simulink model "BLDCmotorControl_FOC_R2017b"  (R2017b)
settings: Solver=FixedStepDiscrete  StartTime=0  StopTime=1  FixedStep=Ts  MaxStep=1e-6  RelTol=1e-6  AbsTol=1e-6  EnableMultiTasking=on
PreLoadFcn:
  | addpath(genpath('01_Libraries'));
  | addpath(genpath('02_Figures'));
InitFcn:
  | init_model;
values from neighbouring files (symbols this model uses):
  a_elecAngle = 60    [init_model_Ffwd.m]
  a_elecPeriod = 360    [init_model_Ffwd.m]
  b_DCLinkCurrAvail = 0    [init_model_Ffwd.m]
  b_selPhaABCurrMeas = 1    [init_model_Ffwd.m]
  cf_speedCoef = round(f_ctrl * a_mechAngle * (pi/180) * (30/pi))    [init_model_Ffwd.m]
  i_thresOutlier = 200    [init_model_Ffwd.m]
  n_commAcvLo = 15    [init_model_Ffwd.m]
  n_commDeacvHi = 30    [init_model_Ffwd.m]
  r_sin_M1 = sin((a_elecAngle_XA + 30)*(pi/180))    [init_model_Ffwd.m]
  r_whl = 6.5 * 2.54 * 1e-2 / 2    (= 0.08255)    [init_model_Ffwd.m]
  res_elecAngle = 2    [init_model_Ffwd.m]
  Ts = 5e-6    (= 5e-06)    [init_model_Ffwd.m]    (also in pe_electric_engine_dyno_data.m = 1e-05)
  Ts_ctrl = 6e-5    (= 6e-05)    [init_model_Ffwd.m]
  vec_hallToPos = [0 2 0 1 4 3 5 0]    [init_model_Ffwd.m]
  z_commutMap_M1 = [-1 -1  0  1  1  0 ... (first row only)    [init_model_Ffwd.m]
  z_ctrlTypSel = 1    [init_model_Ffwd.m]
  z_maxCntRst = 2000    [init_model_Ffwd.m]
undefined symbols (not defined in the file or in its folder): a_phaAdv_M1, b_phaAdvEna, CTRL_COMM, DiscIntNeverNeededParam, Down, dz_counterHi, dz_counterLo, Kb_Id, Kb_Iq, Kb_n, Ki_Id, Ki_Iq, Ki_n, Kp_Id, Kp_Iq, Kp_n, n_motPhaAdvEna, r_commDCDeacv, sigbuilder_block, Up, V_circleLim_M1, V_max, V_min
libraries: pePwmGenerator x7, BLDC_controller_Lib x6, powerlib x6, simulink x5
(part 2 of 3)

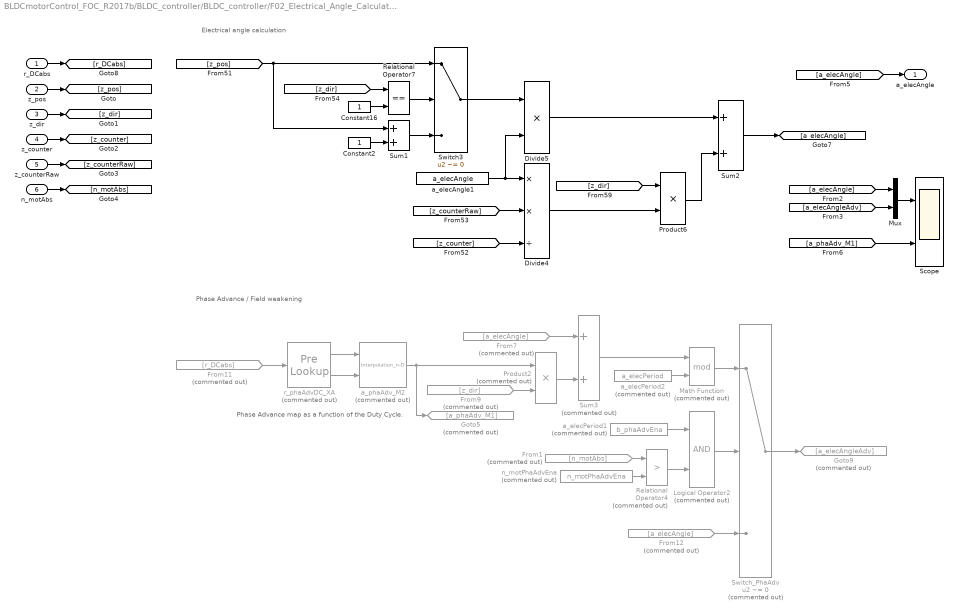
== system BLDCmotorControl_FOC_R2017b/BLDC_controller/BLDC_controller/F02_Electrical_Angle_Calculation ==
  note: Electrical angle calculation
  note: Phase Advance / Field weakening
  note: Phase Advance map as a function of the Duty Cycle.
  r_DCabs : Inport
  z_pos : Inport  Port=2
  z_dir : Inport  Port=3
  z_counter : Inport  Port=4
  z_counterRaw : Inport  Port=5
  n_motAbs : Inport  Port=6
  Constant16 : Constant  OutDataTypeStr=Inherit: Inherit via back propagation
  Constant2 : Constant  OutDataTypeStr=Inherit: Inherit via back propagation
  Divide4 : Product  Inputs=**/  OutDataTypeStr=int32  RndMeth=Simplest
  Divide5 : Product  Inputs=**  OutDataTypeStr=int32  RndMeth=Simplest
  From1 : From  Commented=on  GotoTag=n_motAbs
  From11 : From  Commented=on  GotoTag=r_DCabs
  From12 : From  Commented=on  GotoTag=a_elecAngle
  From7 : From  Commented=on  GotoTag=a_elecAngle
  From9 : From  Commented=on  GotoTag=z_dir
  Goto5 : Goto  Commented=on  GotoTag=a_phaAdv_M1
  Goto9 : Goto  Commented=on  GotoTag=a_elecAngleAdv
  Logical Operator2 : Logic  Commented=on  AllPortsSameDT=off  OutDataTypeStr=boolean
  Math Function : Math  Commented=on  Operator=mod  SaturateOnIntegerOverflow=on
  Mux : Mux  Inputs=2
  Product2 : Product  Commented=on  RndMeth=Simplest  OutDataTypeStr=Inherit: Same as first input
  Product6 : Product  OutDataTypeStr=Inherit: Inherit via back propagation  RndMeth=Simplest
  Relational Operator4 : RelationalOperator  Commented=on  Operator=>  OutDataTypeStr=boolean  RndMeth=Simplest
  Relational Operator7 : RelationalOperator  Operator===  OutDataTypeStr=boolean  RndMeth=Simplest
  Scope : Scope  NumInputPorts=2
  Sum1 : Sum  RndMeth=Simplest  OutDataTypeStr=Inherit: Same as first input
  Sum2 : Sum  RndMeth=Simplest  OutDataTypeStr=Inherit: Same as first input
  Sum3 : Sum  Commented=on  RndMeth=Simplest  OutDataTypeStr=Inherit: Same as first input
  Switch3 : Switch  Criteria=u2 ~= 0  OutDataTypeStr=Inherit: Inherit via back propagation  RndMeth=Zero
  Switch_PhaAdv : Switch  Commented=on  Criteria=u2 ~= 0  OutDataTypeStr=Inherit: Inherit via back propagation  RndMeth=Zero
  a_elecAngle1 : Constant  Value=a_elecAngle  OutDataTypeStr=int32
  a_elecPeriod1 : Constant  Commented=on  Value=b_phaAdvEna  OutDataTypeStr=boolean
  a_elecPeriod2 : Constant  Commented=on  Value=a_elecPeriod  OutDataTypeStr=Inherit: Inherit via back propagation
  a_phaAdv_M2 : Interpolation_n-D  Commented=on  NumberOfTableDimensions=1  Table=a_phaAdv_M1  ExtrapMethod=Clip  OutDataTypeStr=int16  InternalRulePriority=Speed  RndMeth=Simplest
      settings: InputPortMap=u0,u1
  n_motPhaAdvEna : Constant  Commented=on  Value=n_motPhaAdvEna  OutDataTypeStr=Inherit: Inherit via back propagation
  r_phaAdvDC_XA : PreLookup  Commented=on  BreakpointsData=r_phaAdvDC_XA  IndexSearchMethod=Evenly spaced points  BeginIndexSearchUsingPreviousIndexResult=on  IndexDataTypeStr=uint8  RndMeth=Simplest
  a_elecAngle : Outport  OutputWhenDisabled=reset  InitialOutput=0
  wires:
  a_phaAdv_M2/1 -> Goto5/1, Product2/1
  From9/1 -> Product2/2
  z_pos/1 -> [z_pos]
  z_dir/1 -> [z_dir]
  Mux/1 -> Scope/1
  [a_elecAngle] -> Mux/1
  [a_elecAngleAdv] -> Mux/2
  [a_elecAngle] -> a_elecAngle/1
  [a_phaAdv_M1] -> Scope/2
  r_phaAdvDC_XA/2 -> a_phaAdv_M2/2
  r_phaAdvDC_XA/1 -> a_phaAdv_M2/1
  From12/1 -> Switch_PhaAdv/3
  r_DCabs/1 -> [r_DCabs]
  Switch_PhaAdv/1 -> Goto9/1
  Product2/1 -> Sum3/2
  From7/1 -> Sum3/1
  From11/1 -> r_phaAdvDC_XA/1
  a_elecPeriod2/1 -> Math Function/2
  Math Function/1 -> Switch_PhaAdv/1
  Sum3/1 -> Math Function/1
  z_counterRaw/1 -> [z_counterRaw]
  z_counter/1 -> [z_counter]
  [z_counterRaw] -> Divide4/2
  Switch3/1 -> Divide5/1
  [z_dir] -> Product6/1
  Sum2/1 -> [a_elecAngle]
  [z_pos] -> Switch3/1, Sum1/1
  Constant2/1 -> Sum1/2
  [z_counter] -> Divide4/3
  Product6/1 -> Sum2/2
  Relational Operator7/1 -> Switch3/2
  Constant16/1 -> Relational Operator7/2
  a_elecAngle1/1 -> Divide5/2, Divide4/1
  [z_dir] -> Relational Operator7/1
  Sum1/1 -> Switch3/3
  Divide4/1 -> Product6/2
  Divide5/1 -> Sum2/1
  a_elecPeriod1/1 -> Logical Operator2/1
  n_motPhaAdvEna/1 -> Relational Operator4/2
  From1/1 -> Relational Operator4/1
  Relational Operator4/1 -> Logical Operator2/2
  Logical Operator2/1 -> Switch_PhaAdv/2
  n_motAbs/1 -> [n_motAbs]

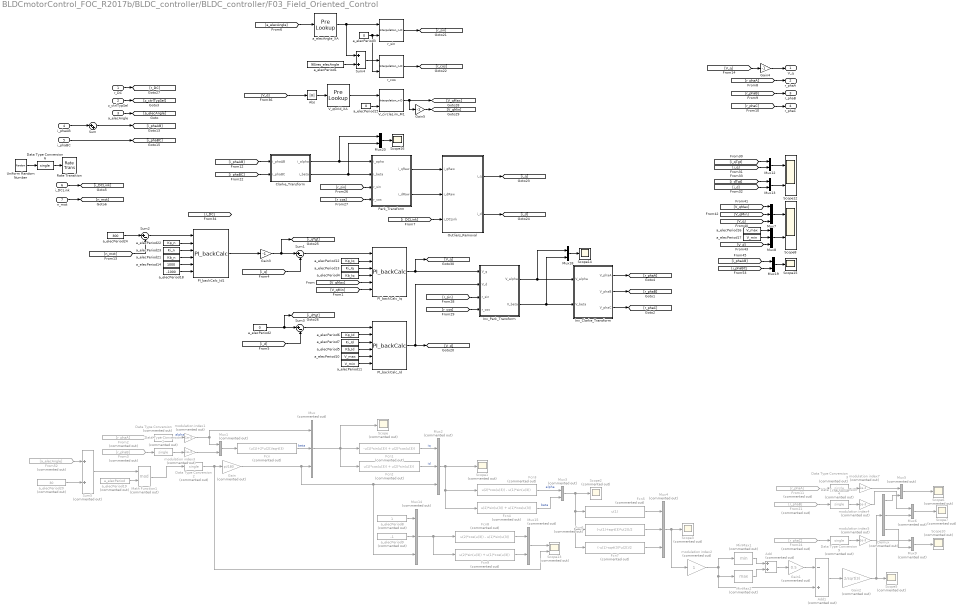
== system BLDCmotorControl_FOC_R2017b/BLDC_controller/BLDC_controller/F03_Field_Oriented_Control ==
  r_DC : Inport
  z_ctrlTypSel : Inport  Port=2
  a_elecAngle : Inport  Port=3
  i_phaAB : Inport  Port=4
  i_phaBC : Inport  Port=5
  i_DCLink : Inport  Port=6
  n_mot : Inport  Port=7
  Abs : Abs
  Add : Sum  Commented=on
  Add1 : Sum  Commented=on  Inputs=-+
  Clarke_Transform : Subsystem
  Data Type Conversion{,1..4,9} (6 alike) : DataTypeConversion  Commented=on  OutDataTypeStr=single
  Data Type Conversion6 : DataTypeConversion  OutDataTypeStr=single
  Demux : Demux  Commented=on  Outputs=3
  Fcn : Fcn  Commented=on  Expr=(u(1)+2*u(2))/sqrt(3)
  Fcn1 : Fcn  Commented=on  Expr=-u(1)*sin(u(3)) + u(2)*cos(u(3))
  Fcn2 : Fcn  Commented=on  Expr=u(1)*cos(u(3)) + u(2)*sin(u(3))
  Fcn3 : Fcn  Commented=on  Expr=u(2)*cos(u(3)) - u(1)*sin(u(3))
  Fcn4 : Fcn  Commented=on  Expr=u(2)*sin(u(3)) + u(1)*cos(u(3))
  Fcn5 : Fcn  Commented=on  Expr=u(1)
  Fcn6 : Fcn  Commented=on  Expr=(-u(1)+sqrt(3)*u(2))/2
  Fcn7 : Fcn  Commented=on  Expr=(-u(1)-sqrt(3)*u(2))/2
  Fcn8 : Fcn  Commented=on  Expr=u(2)*cos(u(3)) - u(1)*sin(u(3))
  Fcn9 : Fcn  Commented=on  Expr=u(2)*sin(u(3)) + u(1)*cos(u(3))
  From11 : From  Commented=on  GotoTag=r_phaA
  From2 : From  Commented=on  GotoTag=r_phaA
  From21 : From  Commented=on  GotoTag=r_phaB
  From24 : From  Commented=on  GotoTag=r_phaC
  From3 : From  Commented=on  GotoTag=r_phaB
  From52 : From  Commented=on  GotoTag=a_elecAngle
  Gain : Gain  Tag=struct('comment',struct('text','','placement',1),'logdata',struct('maxnumvals',inf,'plotchannels',[],'loggingmode',3,'channels',1),'output',struct('variable','','description','','name','$S_$B','width',1,'address','','max',NaN,'min',NaN,'class','default','type','CONTINUOUS','scaling','','lsb',1,'offset',0,'arb',0,'freeze',1,'unit','','autoscalingmode',1,'lowerheadroom',1,'upperheadroom',1,'headroomunit','bit','keepdatatype',1,'checkmin',0,'checkmax',0,'castoutput',0,'show',0),'gain',struct('variable','','description','','name','$S_$B_gain','width',1,'address','','max',NaN,'min',NaN,'class','default','type','CONTINUOUS','scaling','','lsb',1,'offset',0,'arb',0,'freeze',1,'unit','','keepdatatype',1,'value','1','scalar',0,'tolerance',1),'scalingvalid',0,'date',730486)  Commented=on  Gain=pi/180  RndMeth=Zero  SaturateOnIntegerOverflow=on  OutDataTypeStr=Inherit: Same as input  ParamDataTypeStr=Inherit: Same as input
  Gain1 : Gain  Commented=on  Gain=0.5
  Gain2 : Gain  Commented=on  Gain=2/sqrt(3)
  Gain3 : Gain  Tag=struct('comment',struct('text','','placement',1),'logdata',struct('maxnumvals',inf,'plotchannels',[],'loggingmode',3,'channels',1),'output',struct('variable','','description','','name','$S_$B','width',1,'address','','max',NaN,'min',NaN,'class','default','type','CONTINUOUS','scaling','','lsb',1,'offset',0,'arb',0,'freeze',1,'unit','','autoscalingmode',1,'lowerheadroom',1,'upperheadroom',1,'headroomunit','bit','keepdatatype',1,'checkmin',0,'checkmax',0,'castoutput',0,'show',0),'gain',struct('variable','','description','','name','$S_$B_gain','width',1,'address','','max',NaN,'min',NaN,'class','default','type','CONTINUOUS','scaling','','lsb',1,'offset',0,'arb',0,'freeze',1,'unit','','keepdatatype',1,'value','1','scalar',0,'tolerance',1),'scalingvalid',0,'date',730486)  Gain=-1  RndMeth=Zero  SaturateOnIntegerOverflow=on  OutDataTypeStr=Inherit: Same as input  ParamDataTypeStr=Inherit: Same as input
  Gain4 : Gain  Tag=struct('comment',struct('text','','placement',1),'logdata',struct('maxnumvals',inf,'plotchannels',[],'loggingmode',3,'channels',1),'output',struct('variable','','description','','name','$S_$B','width',1,'address','','max',NaN,'min',NaN,'class','default','type','CONTINUOUS','scaling','','lsb',1,'offset',0,'arb',0,'freeze',1,'unit','','autoscalingmode',1,'lowerheadroom',1,'upperheadroom',1,'headroomunit','bit','keepdatatype',1,'checkmin',0,'checkmax',0,'castoutput',0,'show',0),'gain',struct('variable','','description','','name','$S_$B_gain','width',1,'address','','max',NaN,'min',NaN,'class','default','type','CONTINUOUS','scaling','','lsb',1,'offset',0,'arb',0,'freeze',1,'unit','','keepdatatype',1,'value','1','scalar',0,'tolerance',1),'scalingvalid',0,'date',730486)  Gain=-1  RndMeth=Zero  SaturateOnIntegerOverflow=on  OutDataTypeStr=Inherit: Same as input  ParamDataTypeStr=Inherit: Same as input
  Gain5 : Gain  Tag=struct('comment',struct('text','','placement',1),'logdata',struct('maxnumvals',inf,'plotchannels',[],'loggingmode',3,'channels',1),'output',struct('variable','','description','','name','$S_$B','width',1,'address','','max',NaN,'min',NaN,'class','default','type','CONTINUOUS','scaling','','lsb',1,'offset',0,'arb',0,'freeze',1,'unit','','autoscalingmode',1,'lowerheadroom',1,'upperheadroom',1,'headroomunit','bit','keepdatatype',1,'checkmin',0,'checkmax',0,'castoutput',0,'show',0),'gain',struct('variable','','description','','name','$S_$B_gain','width',1,'address','','max',NaN,'min',NaN,'class','default','type','CONTINUOUS','scaling','','lsb',1,'offset',0,'arb',0,'freeze',1,'unit','','keepdatatype',1,'value','1','scalar',0,'tolerance',1),'scalingvalid',0,'date',730486)  Gain=-1  RndMeth=Zero  SaturateOnIntegerOverflow=on  OutDataTypeStr=Inherit: Same as input  ParamDataTypeStr=Inherit: Same as input
  Inv_Clarke_Transform : Subsystem
  Inv_Park_Transform : Subsystem
  Math Function1 : Math  Commented=on  Operator=mod  SaturateOnIntegerOverflow=on
  MinMax1 : MinMax  Commented=on  SaturateOnIntegerOverflow=on  InputSameDT=on
  MinMax2 : MinMax  Commented=on  Function=max  SaturateOnIntegerOverflow=on  InputSameDT=on
  Mux{,2,4,14} (4 alike) : Mux  Commented=on  Inputs=3
  Mux{1,3,5..6,9,15} (6 alike) : Mux  Commented=on  Inputs=2
  Mux{12..13,18..20} (5 alike) : Mux  Inputs=2
  Mux7 : Mux  Inputs=3
  Mux8 : Mux  Inputs=3
  Outliers_Removal : Subsystem
  PI_backCalc_Id : BLDC_controller_Lib/PI_backCalc  SystemSampleTime=-1
  PI_backCalc_Id1 : BLDC_controller_Lib/PI_backCalc  SystemSampleTime=-1
  PI_backCalc_Iq : BLDC_controller_Lib/PI_backCalc  SystemSampleTime=-1
  Park_Transform : Subsystem
  Rate Transition : RateTransition
  Scope{,1..3,5..7,10} (8 alike) : Scope  Commented=on
  Scope12 : Scope  NumInputPorts=2
  Scope13 : Scope  Commented=on  NumInputPorts=2
  Scope14 : Scope
  Scope15 : Scope
  Scope16 : Scope
  Scope8 : Scope  NumInputPorts=2
  Sum : Sum  Inputs=|++
  Sum1 : Sum  Inputs=|+-  RndMeth=Simplest  OutDataTypeStr=Inherit: Same as first input
  Sum2 : Sum  Inputs=|+-  RndMeth=Simplest  OutDataTypeStr=Inherit: Same as first input
  Sum3 : Sum  Inputs=|+-  RndMeth=Simplest  OutDataTypeStr=Inherit: Same as first input
  Sum4 : Sum  RndMeth=Simplest  OutDataTypeStr=Inherit: Same as first input
  Sum5 : Sum  Commented=on  RndMeth=Simplest  OutDataTypeStr=Inherit: Same as first input
  Uniform Random Number : UniformRandomNumber  Minimum=-1000  Maximum=1000  SampleTime=6e-05  VectorParams1D=off
  V_circleLim_M1 : Interpolation_n-D  NumberOfTableDimensions=1  Table=V_circleLim_M1  InterpMethod=Flat  ExtrapMethod=Clip  ValidIndexMayReachLast=on  OutDataTypeStr=single  InternalRulePriority=Speed  RndMeth=Simplest
      settings: InputPortMap=u0,u1
  V_qGrid_XA : PreLookup  BreakpointsData=V_qGrid_XA  OutputSelection=Index only  IndexSearchMethod=Evenly spaced points  BeginIndexSearchUsingPreviousIndexResult=on  IndexDataTypeStr=uint8  RndMeth=Simplest
  a_elecAngle_XA : PreLookup  BreakpointsData=a_elecAngle_XA  OutputSelection=Index only  IndexSearchMethod=Evenly spaced points  BeginIndexSearchUsingPreviousIndexResult=on  IndexDataTypeStr=uint8  RndMeth=Simplest
  a_elecPeriod1 : Constant  Value=90/res_elecAngle  OutDataTypeStr=uint8
  a_elecPeriod10 : Constant  Value=V_max  OutDataTypeStr=Inherit: Inherit via back propagation
  a_elecPeriod11 : Constant  Value=V_min  OutDataTypeStr=Inherit: Inherit via back propagation
  a_elecPeriod12 : Constant  Value=Kp_Iq  OutDataTypeStr=Inherit: Inherit via back propagation
  a_elecPeriod13 : Constant  Value=Ki_Iq  OutDataTypeStr=Inherit: Inherit via back propagation
  a_elecPeriod14 : Constant  Value=1000  OutDataTypeStr=Inherit: Inherit via back propagation
  a_elecPeriod15 : Constant  Value=0  OutDataTypeStr=uint8
  a_elecPeriod16 : Constant  Value=V_max  OutDataTypeStr=Inherit: Inherit via back propagation
  a_elecPeriod17 : Constant  Value=V_min  OutDataTypeStr=Inherit: Inherit via back propagation
  a_elecPeriod18 : Constant  Value=-1000  OutDataTypeStr=Inherit: Inherit via back propagation
  a_elecPeriod19 : Constant  Commented=on  Value=a_elecPeriod  OutDataTypeStr=Inherit: Inherit via back propagation
  a_elecPeriod2 : Constant  Value=0  OutDataTypeStr=Inherit: Inherit via back propagation
  a_elecPeriod20 : Constant  Commented=on  Value=30  OutDataTypeStr=Inherit: Inherit via back propagation
  a_elecPeriod21 : Constant  Value=Kb_n  OutDataTypeStr=Inherit: Inherit via back propagation
  a_elecPeriod22 : Constant  Value=Kp_n  OutDataTypeStr=Inherit: Inherit via back propagation
  a_elecPeriod23 : Constant  Value=Ki_n  OutDataTypeStr=Inherit: Inherit via back propagation
  a_elecPeriod24 : Constant  Value=300  OutDataTypeStr=Inherit: Inherit via back propagation
  a_elecPeriod3 : Constant  Value=0  OutDataTypeStr=uint8
  a_elecPeriod4 : Constant  Value=Kb_Iq  OutDataTypeStr=Inherit: Inherit via back propagation
  a_elecPeriod5 : Constant  Value=Kb_Id  OutDataTypeStr=Inherit: Inherit via back propagation
  a_elecPeriod6 : Constant  Value=Kp_Id  OutDataTypeStr=Inherit: Inherit via back propagation
  a_elecPeriod7 : Constant  Value=Ki_Id  OutDataTypeStr=Inherit: Inherit via back propagation
  a_elecPeriod8 : Constant  Commented=on  OutDataTypeStr=Inherit: Inherit via back propagation
  a_elecPeriod9 : Constant  Commented=on  Value=-1  OutDataTypeStr=Inherit: Inherit via back propagation
  modulation index{1,3..5,7} (5 alike) : Gain  Commented=on  Gain=1e-3  SaturateOnIntegerOverflow=on  OutDataTypeStr=Inherit: Same as input  ParamDataTypeStr=Inherit: Same as input
  modulation index2 : Gain  Commented=on  SaturateOnIntegerOverflow=on  OutDataTypeStr=Inherit: Same as input  ParamDataTypeStr=Inherit: Same as input
  r_cos : Interpolation_n-D  NumberOfTableDimensions=1  Table=r_sin_M1  InterpMethod=Flat  ExtrapMethod=Clip  ValidIndexMayReachLast=on  OutDataTypeStr=single  InternalRulePriority=Speed  RndMeth=Simplest
      settings: InputPortMap=u0,u1
  r_sin : Interpolation_n-D  NumberOfTableDimensions=1  Table=r_sin_M1  InterpMethod=Flat  ExtrapMethod=Clip  ValidIndexMayReachLast=on  OutDataTypeStr=single  InternalRulePriority=Speed  RndMeth=Simplest
      settings: InputPortMap=u0,u1
  V_q : Outport  OutputWhenDisabled=reset  InitialOutput=0
  r_phaA : Outport  Port=2  OutputWhenDisabled=reset  InitialOutput=0
  r_phaB : Outport  Port=3  OutputWhenDisabled=reset  InitialOutput=0
  "r_phaC " : Outport  Port=4  OutputWhenDisabled=reset  InitialOutput=0
  wires:
  [r_phaA] -> r_phaA/1
  [r_phaB] -> r_phaB/1
  [r_phaC] -> "r_phaC "/1
  a_elecAngle/1 -> [a_elecAngle]
  z_ctrlTypSel/1 -> [z_ctrlTypSel]
  Data Type Conversion4/1 -> modulation index4/1
  Demux/2 -> Mux6/2
  modulation index3/1 -> Mux1/2
  modulation index1/1 -> Mux/1, Mux1/1
  MinMax1/1 -> Add/1
  modulation index2/1 -> MinMax1/1, Add1/2, MinMax2/1
  Mux/1 -> Scope/1, Fcn1/1, Fcn2/1
  From11/1 -> Data Type Conversion3/1
  Data Type Conversion3/1 -> modulation index7/1
  From21/1 -> Data Type Conversion4/1
  Fcn/1 -> Mux/2  "beta"
  Gain2/1 -> Demux/1, Scope5/1
  Mux4/1 -> modulation index2/1, Scope3/1
  Fcn6/1 -> Mux4/2
  MinMax2/1 -> Add/2
  Mux1/1 -> Fcn/1
  Gain1/1 -> Add1/1
  Fcn5/1 -> Mux4/1
  Data Type Conversion/1 -> modulation index1/1  "alpha"
  Data Type Conversion2/1 -> Scope13/2, Gain/1
  Fcn7/1 -> Mux4/3
  Mux3/1 -> Fcn7/1, Fcn6/1, Fcn5/1, Scope2/1
  Mux5/1 -> Scope6/1
  Gain/1 -> Mux14/3, Mux2/3, Mux/3
  Data Type Conversion1/1 -> modulation index3/1
  Add1/1 -> Gain2/1
  Fcn4/1 -> Mux3/2  "beta"
  Demux/1 -> Mux5/2
  Mux6/1 -> Scope7/1
  Mux2/1 -> Fcn4/1, Fcn3/1, Scope1/1
  Fcn3/1 -> Mux3/1  "alpha"
  Add/1 -> Gain1/1
  a_elecPeriod2/1 -> [i_dTgt], Sum3/1
  Sum1/1 -> PI_backCalc_Iq/1
  Inv_Park_Transform/1(V_alpha) -> Mux18/1, Inv_Clarke_Transform/1(V_alpha)
  Inv_Park_Transform/2(V_beta) -> Mux18/2, Inv_Clarke_Transform/2(V_beta)
  i_phaBC/1 -> [i_phaBC]
  Inv_Clarke_Transform/1(V_phaA) -> [r_phaA]
  Inv_Clarke_Transform/2(V_phaB) -> [r_phaB]
  Inv_Clarke_Transform/3(V_phaC) -> [r_phaC]
  Demux/3 -> Mux9/2
  From24/1 -> Data Type Conversion9/1
  Data Type Conversion9/1 -> modulation index5/1
  Mux9/1 -> Scope10/1
  Fcn1/1 -> Mux2/1  "iq"
  Fcn2/1 -> Mux2/2  "id"
  Mux12/1 -> Scope12/1
  Mux13/1 -> Scope12/2
  Gain3/1 -> Sum1/1, [i_qTgt]
  modulation index7/1 -> Mux5/1
  modulation index4/1 -> Mux6/1
  modulation index5/1 -> Mux9/1
  Math Function1/1 -> Data Type Conversion2/1
  Mux14/1 -> Fcn9/1, Fcn8/1
  a_elecPeriod8/1 -> Mux14/1
  a_elecPeriod9/1 -> Mux14/2
  Fcn8/1 -> Mux15/1
  Fcn9/1 -> Mux15/2
  Mux15/1 -> Scope13/1
  PI_backCalc_Iq/1 -> [V_q], Inv_Park_Transform/1(V_q)
  [V_qMin] -> PI_backCalc_Iq/6
  PI_backCalc_Id/1 -> Inv_Park_Transform/2(V_d), [V_d]
  a_elecAngle_XA/1 -> Sum4/1, r_sin/1
  a_elecPeriod3/1 -> r_cos/2, r_sin/2
  r_sin/1 -> [r_sin]
  r_cos/1 -> [r_cos]
  [r_sin] -> Park_Transform/3(r_sin)
  [r_cos] -> Park_Transform/4(r_cos)
  [r_sin] -> Inv_Park_Transform/3(r_sin)
  [r_cos] -> Inv_Park_Transform/4(r_cos)
  [i_qTgt] -> Mux12/1
  [i_q] -> Mux12/2
  [i_d] -> Mux13/2
  [i_dTgt] -> Mux13/1
  r_DC/1 -> [r_DC]
  a_elecPeriod6/1 -> PI_backCalc_Id/2
  a_elecPeriod7/1 -> PI_backCalc_Id/3
  a_elecPeriod10/1 -> PI_backCalc_Id/5
  Sum3/1 -> PI_backCalc_Id/1
  a_elecPeriod12/1 -> PI_backCalc_Iq/2
  a_elecPeriod13/1 -> PI_backCalc_Iq/3
  [i_phaBC] -> Clarke_Transform/2(i_phaBC)
  Sum4/1 -> r_cos/1
  a_elecPeriod1/1 -> Sum4/2
  V_qGrid_XA/1 -> V_circleLim_M1/1
  a_elecPeriod15/1 -> V_circleLim_M1/2
  V_circleLim_M1/1 -> [V_qMax], Gain5/1
  Gain5/1 -> [V_qMin]
  [V_qMax] -> PI_backCalc_Iq/5
  Mux7/1 -> Scope8/1
  [V_qMax] -> Mux7/1
  [V_q] -> Mux7/3
  [V_qMin] -> Mux7/2
  Mux8/1 -> Scope8/2
  [V_d] -> Mux8/3
  a_elecPeriod16/1 -> Mux8/1
  a_elecPeriod17/1 -> Mux8/2
  Abs/1 -> V_qGrid_XA/1
  [a_elecAngle] -> a_elecAngle_XA/1
  a_elecPeriod20/1 -> Sum5/2
  From52/1 -> Sum5/1
  Sum5/1 -> Math Function1/1
  a_elecPeriod19/1 -> Math Function1/2
  Mux18/1 -> Scope14/1
  Mux19/1 -> Scope15/1
  [i_phaBC] -> Mux19/2
  [i_phaAB] -> Mux19/1
  From2/1 -> Data Type Conversion/1
  From3/1 -> Data Type Conversion1/1
  Mux20/1 -> Scope16/1
  a_elecPeriod11/1 -> PI_backCalc_Id/6
  [i_phaAB] -> Clarke_Transform/1(i_phaAB)
  i_phaAB/1 -> Sum/1
  Uniform Random Number/1 -> Data Type Conversion6/1
  Sum/1 -> [i_phaAB]
  Data Type Conversion6/1 -> Rate Transition/1
  Clarke_Transform/1(i_alpha) -> Mux20/1, Park_Transform/1(i_apha)
  Clarke_Transform/2(i_beta) -> Mux20/2, Park_Transform/2(i_beta)
  [i_q] -> Sum1/2
  [i_d] -> Sum3/2
  a_elecPeriod4/1 -> PI_backCalc_Iq/4
  a_elecPeriod5/1 -> PI_backCalc_Id/4
  Park_Transform/1(i_qRaw) -> Outliers_Removal/1(i_qRaw)
  Park_Transform/2(i_dRaw) -> Outliers_Removal/2(i_dRaw)
  Outliers_Removal/2(i_d) -> [i_d]
  Outliers_Removal/1(i_q) -> [i_q]
  i_DCLink/1 -> [i_DCLink]
  [i_DCLink] -> Outliers_Removal/3(i_DCLink)
  [V_d] -> Abs/1
  [V_q] -> Gain4/1
  Gain4/1 -> V_q/1
  a_elecPeriod21/1 -> PI_backCalc_Id1/4
  a_elecPeriod18/1 -> PI_backCalc_Id1/6
  Sum2/1 -> PI_backCalc_Id1/1
  a_elecPeriod14/1 -> PI_backCalc_Id1/5
  a_elecPeriod23/1 -> PI_backCalc_Id1/3
  a_elecPeriod22/1 -> PI_backCalc_Id1/2
  a_elecPeriod24/1 -> Sum2/1
  n_mot/1 -> [n_mot]
  [n_mot] -> Sum2/2
  PI_backCalc_Id1/1 -> Gain3/1

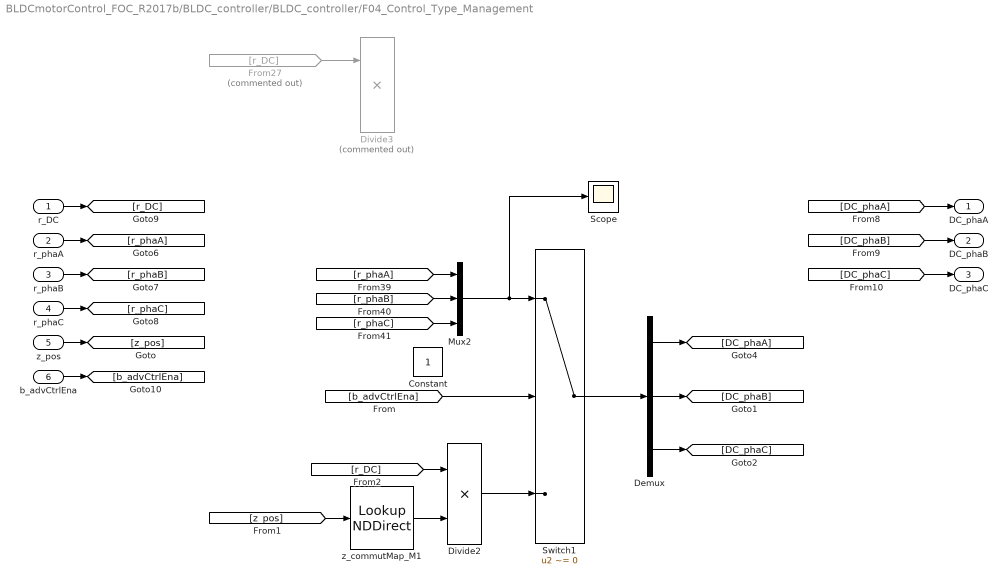
== system BLDCmotorControl_FOC_R2017b/BLDC_controller/BLDC_controller/F04_Control_Type_Management ==
  r_DC : Inport
  r_phaA : Inport  Port=2
  r_phaB : Inport  Port=3
  r_phaC : Inport  Port=4
  z_pos : Inport  Port=5
  b_advCtrlEna : Inport  Port=6
  Constant : Constant  OutDataTypeStr=boolean
  Demux : Demux  Outputs=3
  Divide2 : Product  Inputs=**  RndMeth=Simplest  OutDataTypeStr=Inherit: Same as first input
  Divide3 : Product  Commented=on  Inputs=**  RndMeth=Simplest  OutDataTypeStr=Inherit: Same as first input
  From27 : From  Commented=on  GotoTag=r_DC
  Mux2 : Mux  Inputs=3
  Scope : Scope
  Switch1 : Switch  Criteria=u2 ~= 0  OutDataTypeStr=Inherit: Inherit via back propagation  RndMeth=Zero
  z_commutMap_M1 : LookupNDDirect  InputsSelectThisObjectFromTable=Column  Table=z_commutMap_M1  DiagnosticForOutOfRangeInput=None  TableDataTypeStr=int16
  DC_phaA : Outport  OutputWhenDisabled=reset  InitialOutput=0
  DC_phaB : Outport  Port=2  OutputWhenDisabled=reset  InitialOutput=0
  "DC_phaC " : Outport  Port=3  OutputWhenDisabled=reset  InitialOutput=0
  wires:
  Demux/3 -> [DC_phaC]
  Demux/2 -> [DC_phaB]
  Demux/1 -> [DC_phaA]
  z_pos/1 -> [z_pos]
  [DC_phaC] -> "DC_phaC "/1
  [DC_phaB] -> DC_phaB/1
  [DC_phaA] -> DC_phaA/1
  [z_pos] -> z_commutMap_M1/1
  Switch1/1 -> Demux/1
  r_phaA/1 -> [r_phaA]
  r_phaB/1 -> [r_phaB]
  r_phaC/1 -> [r_phaC]
  r_DC/1 -> [r_DC]
  [r_phaA] -> Mux2/1
  [r_phaB] -> Mux2/2
  [r_phaC] -> Mux2/3
  [r_DC] -> Divide2/1
  z_commutMap_M1/1 -> Divide2/2
  Divide2/1 -> Switch1/3
  b_advCtrlEna/1 -> [b_advCtrlEna]
  From27/1 -> Divide3/1
  Mux2/1 -> Scope/1, Switch1/1
  [b_advCtrlEna] -> Switch1/2

== system BLDCmotorControl_FOC_R2017b/BLDC_controller/BLDC_controller/Implemented_control_methods ==

== system BLDCmotorControl_FOC_R2017b/PWM_gates/PWM_generator1/__InputSSForSFun__ ==
  DC : Inport  SampleTime=Ts
  __UniqueOutportName__1__ : Outport
  wires:
  DC/1 -> __UniqueOutportName__1__/1

== system BLDCmotorControl_FOC_R2017b/PWM_gates/PWM_generator1/__OutputSSForSFun__ ==
  __UniqueInportName__1__ : Inport
  PWM : Outport
  wires:
  __UniqueInportName__1__/1 -> PWM/1

== system BLDCmotorControl_FOC_R2017b/PWM_gates/PWM_generator12/__InputSSForSFun__ ==
  DC : Inport  SampleTime=Ts
  __UniqueOutportName__1__ : Outport
  wires:
  DC/1 -> __UniqueOutportName__1__/1

== system BLDCmotorControl_FOC_R2017b/PWM_gates/PWM_generator12/__OutputSSForSFun__ ==
  __UniqueInportName__1__ : Inport
  PWM : Outport
  wires:
  __UniqueInportName__1__/1 -> PWM/1

== system BLDCmotorControl_FOC_R2017b/PWM_gates/PWM_generator2/__InputSSForSFun__ ==
  DC : Inport  SampleTime=Ts
  __UniqueOutportName__1__ : Outport
  wires:
  DC/1 -> __UniqueOutportName__1__/1

== system BLDCmotorControl_FOC_R2017b/PWM_gates/PWM_generator2/__OutputSSForSFun__ ==
  __UniqueInportName__1__ : Inport
  PWM : Outport
  wires:
  __UniqueInportName__1__/1 -> PWM/1

== system BLDCmotorControl_FOC_R2017b/PWM_gates/PWM_generator3/__InputSSForSFun__ ==
  DC : Inport  SampleTime=Ts
  __UniqueOutportName__1__ : Outport
  wires:
  DC/1 -> __UniqueOutportName__1__/1

== system BLDCmotorControl_FOC_R2017b/PWM_gates/PWM_generator3/__OutputSSForSFun__ ==
  __UniqueInportName__1__ : Inport
  PWM : Outport
  wires:
  __UniqueInportName__1__/1 -> PWM/1

== system BLDCmotorControl_FOC_R2017b/PWM_gates/PWM_generator4/__InputSSForSFun__ ==
  DC : Inport  SampleTime=Ts
  __UniqueOutportName__1__ : Outport
  wires:
  DC/1 -> __UniqueOutportName__1__/1

== system BLDCmotorControl_FOC_R2017b/PWM_gates/PWM_generator4/__OutputSSForSFun__ ==
  __UniqueInportName__1__ : Inport
  PWM : Outport
  wires:
  __UniqueInportName__1__/1 -> PWM/1

== system BLDCmotorControl_FOC_R2017b/PWM_gates/PWM_generator5/__InputSSForSFun__ ==
  DC : Inport  SampleTime=Ts
  __UniqueOutportName__1__ : Outport
  wires:
  DC/1 -> __UniqueOutportName__1__/1

== system BLDCmotorControl_FOC_R2017b/PWM_gates/PWM_generator5/__OutputSSForSFun__ ==
  __UniqueInportName__1__ : Inport
  PWM : Outport
  wires:
  __UniqueInportName__1__/1 -> PWM/1

== system BLDCmotorControl_FOC_R2017b/BLDC_controller/BLDC_controller/F01_Preliminary_Calculations/F01_01_Edge_Detector ==
  b_hallA : Inport
  b_hallB : Inport  Port=2
  b_hallC : Inport  Port=3
  Bitwise Operator : simulink/Logic and Bit Operations/Bitwise Operator  logicop=XOR  UseBitMask=off  NumInputPorts=6  BitMask=bin2dec('11011001')  BitMaskRealWorld=Stored Integer
  UnitDelay : UnitDelay  SampleTime=-1
  UnitDelay1 : UnitDelay  SampleTime=-1
  UnitDelay2 : UnitDelay  SampleTime=-1
  "b_edge " : Outport  OutputWhenDisabled=reset  InitialOutput=0
  wires:
  b_hallA/1 -> Bitwise Operator/1, UnitDelay/1
  b_hallC/1 -> Bitwise Operator/3, UnitDelay2/1
  b_hallB/1 -> Bitwise Operator/2, UnitDelay1/1
  Bitwise Operator/1 -> "b_edge "/1
  UnitDelay1/1 -> Bitwise Operator/5
  UnitDelay2/1 -> Bitwise Operator/6
  UnitDelay/1 -> Bitwise Operator/4

== system BLDCmotorControl_FOC_R2017b/BLDC_controller/BLDC_controller/F01_Preliminary_Calculations/F01_02_Position_Calculation ==
  note: This calculates the low resolution position based on Hall sensors.
  b_hallA : Inport
  b_hallB : Inport  Port=2
  b_hallC : Inport  Port=3
  Selector : Selector  IndexMode=Zero-based  InputPortWidth=length(vec_hallToPos)  IndexOptions=Index vector (port)  Indices=[1 3]  OutputSizes=1
  Sum : Sum  Inputs=+++  RndMeth=Simplest  OutDataTypeStr=Inherit: Same as first input
  g_Ha : Gain  Gain=4  OutDataTypeStr=Inherit: Inherit via back propagation  RndMeth=Zero  ParamDataTypeStr=Inherit: Same as input
  g_Hb : Gain  Gain=2  OutDataTypeStr=Inherit: Inherit via back propagation  RndMeth=Simplest  ParamDataTypeStr=Inherit: Same as input
  vec_hallToPos : Constant  Value=vec_hallToPos  OutDataTypeStr=int8
  "z_pos " : Outport  OutputWhenDisabled=reset  InitialOutput=0
  wires:
  b_hallC/1 -> Sum/3
  g_Ha/1 -> Sum/1
  g_Hb/1 -> Sum/2
  Sum/1 -> Selector/2
  b_hallA/1 -> g_Ha/1
  b_hallB/1 -> g_Hb/1
  vec_hallToPos/1 -> Selector/1
  Selector/1 -> "z_pos "/1

== system BLDCmotorControl_FOC_R2017b/BLDC_controller/BLDC_controller/F01_Preliminary_Calculations/F01_03_Direction_Detection ==
  z_pos : Inport
  Action Port : ActionPort  ActionType=then
  Constant20 : Constant  Value=-5  OutDataTypeStr=Inherit: Inherit via back propagation
  Constant23 : Constant  Value=-1  OutDataTypeStr=int8
  Constant24 : Constant  OutDataTypeStr=int8
  Constant8 : Constant  OutDataTypeStr=Inherit: Inherit via back propagation
  Logical Operator3 : Logic  Operator=OR  AllPortsSameDT=off  OutDataTypeStr=boolean
  Relational Operator1 : RelationalOperator  Operator===  OutDataTypeStr=boolean  RndMeth=Simplest
  Relational Operator6 : RelationalOperator  Operator===  OutDataTypeStr=boolean  RndMeth=Simplest
  Sum2 : Sum  Inputs=|+-  RndMeth=Zero  InputSameDT=on  OutDataTypeStr=Inherit: Same as first input
  Switch2 : Switch  Criteria=u2 ~= 0  OutDataTypeStr=Inherit: Inherit via back propagation  RndMeth=Simplest
  UnitDelay1 : UnitDelay  SampleTime=-1
  UnitDelay2 : UnitDelay  SampleTime=-1
  z_dir : Outport
  z_dirPrev : Outport  Port=2
  wires:
  UnitDelay2/1 -> Sum2/2
  Relational Operator1/1 -> Logical Operator3/1
  Constant8/1 -> Relational Operator1/2
  Sum2/1 -> Relational Operator6/1, Relational Operator1/1
  Relational Operator6/1 -> Logical Operator3/2
  Constant20/1 -> Relational Operator6/2
  Constant24/1 -> Switch2/1
  Constant23/1 -> Switch2/3
  Logical Operator3/1 -> Switch2/2
  z_pos/1 -> Sum2/1, UnitDelay2/1
  Switch2/1 -> UnitDelay1/1, z_dir/1
  UnitDelay1/1 -> z_dirPrev/1

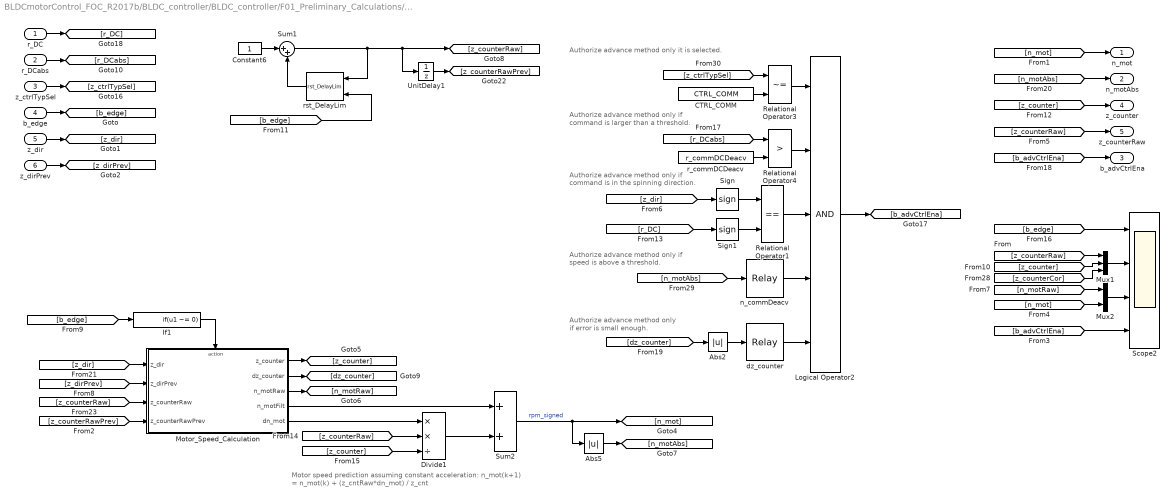
== system BLDCmotorControl_FOC_R2017b/BLDC_controller/BLDC_controller/F01_Preliminary_Calculations/F01_04_Speed_Calculation ==
  note: Authorize advance method only if speed is above a threshold.
  note: Authorize advance method only if command is in the spinning direction.
  note: Authorize advance method only if error is small enough.
  note: Authorize advance method only if command is larger than a threshold.
  note: Authorize advance method only it is selected.
  note: Motor speed prediction assuming constant acceleration:
      | n_mot(k+1) = n_mot(k) + (z_cntRaw*dn_mot) / z_cnt
  r_DC : Inport
  r_DCabs : Inport  Port=2
  z_ctrlTypSel : Inport  Port=3
  b_edge : Inport  Port=4
  z_dir : Inport  Port=5
  z_dirPrev : Inport  Port=6
  Abs2 : Abs  OutDataTypeStr=Inherit: Inherit via back propagation  RndMeth=Zero
  Abs5 : Abs  OutDataTypeStr=Inherit: Inherit via back propagation  RndMeth=Zero
  CTRL_COMM : Constant  Value=CTRL_COMM  OutDataTypeStr=Inherit: Inherit via back propagation
  Constant6 : Constant  OutDataTypeStr=int16
  Divide1 : Product  Inputs=**/  RndMeth=Simplest  OutDataTypeStr=Inherit: Same as first input
  If1 : If  IfExpression=u1 ~= 0  ShowElse=off
  Logical Operator2 : Logic  Inputs=5  AllPortsSameDT=off  OutDataTypeStr=boolean
  Motor_Speed_Calculation : Subsystem
  Mux1 : Mux  Inputs=3
  Mux2 : Mux  Inputs=2
  Relational Operator1 : RelationalOperator  Operator===  OutDataTypeStr=boolean  RndMeth=Simplest
  Relational Operator3 : RelationalOperator  Operator=~=  OutDataTypeStr=boolean  RndMeth=Simplest
  Relational Operator4 : RelationalOperator  Operator=>  OutDataTypeStr=boolean  RndMeth=Simplest
  Scope2 : Scope  NumInputPorts=4
  Sign : Signum
  Sign1 : Signum
  Sum1 : Sum  Inputs=|++  RndMeth=Simplest  InputSameDT=on  OutDataTypeStr=Inherit: Same as first input
  Sum2 : Sum  RndMeth=Simplest  InputSameDT=on  OutDataTypeStr=Inherit: Same as first input
  UnitDelay1 : UnitDelay  SampleTime=-1
  dz_counter : Relay  OnSwitchValue=dz_counterHi  OffSwitchValue=dz_counterLo  OnOutputValue=0  OffOutputValue=1  OutDataTypeStr=boolean
  n_commDeacv : Relay  OnSwitchValue=n_commDeacvHi  OffSwitchValue=n_commAcvLo  OutDataTypeStr=boolean
  r_commDCDeacv : Constant  Value=r_commDCDeacv  OutDataTypeStr=Inherit: Inherit via back propagation
  rst_DelayLim : BLDC_controller_Lib/rst_DelayLim  z_cntMaxLim=z_maxCntRst
  n_mot : Outport
  n_motAbs : Outport  Port=2
  b_advCtrlEna : Outport  Port=3
  z_counter : Outport  Port=4  OutputWhenDisabled=reset  InitialOutput=0
  z_counterRaw : Outport  Port=5  OutputWhenDisabled=reset  InitialOutput=0
  wires:
  Abs2/1 -> dz_counter/1
  dz_counter/1 -> Logical Operator2/5
  [n_mot] -> Mux2/2
  Mux2/1 -> Scope2/3
  [n_motRaw] -> Mux2/1
  Mux1/1 -> Scope2/2
  [z_counterRaw] -> Mux1/1
  [z_counter] -> Mux1/2
  [b_edge] -> Scope2/1
  Constant6/1 -> Sum1/1
  Sum1/1 -> rst_DelayLim/1, [z_counterRaw], UnitDelay1/1
  b_edge/1 -> [b_edge]
  [n_mot] -> n_mot/1
  z_dir/1 -> [z_dir]
  rst_DelayLim/1 -> Sum1/2
  [z_ctrlTypSel] -> Relational Operator3/1
  [n_motAbs] -> n_commDeacv/1
  CTRL_COMM/1 -> Relational Operator3/2
  [r_DCabs] -> Relational Operator4/1
  r_commDCDeacv/1 -> Relational Operator4/2
  Logical Operator2/1 -> [b_advCtrlEna]
  If1/1 -> Motor_Speed_Calculation/Action
  Motor_Speed_Calculation/1(z_counter) -> [z_counter]
  [z_counterRawPrev] -> Motor_Speed_Calculation/4(z_counterRawPrev)
  Motor_Speed_Calculation/2(dz_counter) -> [dz_counter]
  [dz_counter] -> Abs2/1
  z_ctrlTypSel/1 -> [z_ctrlTypSel]
  r_DC/1 -> [r_DC]
  [b_advCtrlEna] -> b_advCtrlEna/1
  [z_counter] -> z_counter/1
  [z_counterRaw] -> z_counterRaw/1
  [b_edge] -> rst_DelayLim/2
  UnitDelay1/1 -> [z_counterRawPrev]
  [b_advCtrlEna] -> Scope2/4
  [z_dir] -> Sign/1
  Sign/1 -> Relational Operator1/1
  [r_DC] -> Sign1/1
  Sign1/1 -> Relational Operator1/2
  [b_edge] -> If1/1
  z_dirPrev/1 -> [z_dirPrev]
  n_commDeacv/1 -> Logical Operator2/4
  Relational Operator3/1 -> Logical Operator2/1
  Relational Operator4/1 -> Logical Operator2/2
  Relational Operator1/1 -> Logical Operator2/3
  r_DCabs/1 -> [r_DCabs]
  [n_motAbs] -> n_motAbs/1
  [z_dir] -> Motor_Speed_Calculation/1(z_dir)
  Motor_Speed_Calculation/3(n_motRaw) -> [n_motRaw]
  [z_dirPrev] -> Motor_Speed_Calculation/2(z_dirPrev)
  [z_counterRaw] -> Motor_Speed_Calculation/3(z_counterRaw)
  Abs5/1 -> [n_motAbs]
  Divide1/1 -> Sum2/2
  Motor_Speed_Calculation/5(dn_mot) -> Divide1/1
  [z_counterRaw] -> Divide1/2
  [z_counter] -> Divide1/3
  [z_counterCor] -> Mux1/3
  Motor_Speed_Calculation/4(n_motFilt) -> Sum2/1
  Sum2/1 -> [n_mot], Abs5/1  "rpm_signed"

== system BLDCmotorControl_FOC_R2017b/BLDC_controller/BLDC_controller/F03_Field_Oriented_Control/Clarke_Transform ==
  i_phaAB : Inport
  i_phaBC : Inport  Port=2
  Clarke_PhasesAB : Subsystem
  Clarke_PhasesBC : Subsystem
  If1 : If  IfExpression=u1 ~= 0
  Merge : Merge
  Merge1 : Merge
  b_selPhaABCurrMeas : Constant  Value=b_selPhaABCurrMeas  OutDataTypeStr=boolean
  i_alpha : Outport
  i_beta : Outport  Port=2
  wires:
  i_phaAB/1 -> [i_phaAB]
  i_phaBC/1 -> [i_phaBC]
  If1/2 -> Clarke_PhasesBC/Action
  If1/1 -> Clarke_PhasesAB/Action
  b_selPhaABCurrMeas/1 -> If1/1
  Merge/1 -> [i_alpha]
  Merge1/1 -> [i_beta]
  Clarke_PhasesAB/1(i_alphaAB) -> [i_alphaAB]
  Clarke_PhasesBC/1(i_alphaBC) -> [i_alphaBC]
  Clarke_PhasesAB/2(i_betaAB) -> [i_betaAB]
  Clarke_PhasesBC/2(i_betaBC) -> [i_betaBC]
  [i_alphaAB] -> Merge/1
  [i_alphaBC] -> Merge/2
  [i_betaAB] -> Merge1/1
  [i_betaBC] -> Merge1/2
  [i_alpha] -> i_alpha/1
  [i_beta] -> i_beta/1
  [i_phaAB] -> Clarke_PhasesAB/1(i_phaA)
  [i_phaAB] -> Clarke_PhasesBC/1(i_phaB)
  [i_phaBC] -> Clarke_PhasesAB/2(i_phaB)
  [i_phaBC] -> Clarke_PhasesBC/2(i_phaC)

== system BLDCmotorControl_FOC_R2017b/BLDC_controller/BLDC_controller/F03_Field_Oriented_Control/Inv_Clarke_Transform ==
  note: Inverse Clarke Transform:
      | V_phaA = V_alpha
      | V_phaB = -(1/2)*V_alpha + (sqrt(3)/2)*V_beta
      | V_phaC = -VphaA - V_phaB
  V_alpha : Inport
  V_beta : Inport  Port=2
  Add : Sum
  Add1 : Sum  Inputs=-+
  Demux : Demux  Outputs=3
  Gain1 : Gain  Tag=struct('comment',struct('text','','placement',1),'logdata',struct('maxnumvals',inf,'plotchannels',[],'loggingmode',3,'channels',1),'output',struct('variable','','description','','name','$S_$B','width',1,'address','','max',NaN,'min',NaN,'class','default','type','CONTINUOUS','scaling','','lsb',1,'offset',0,'arb',0,'freeze',1,'unit','','autoscalingmode',1,'lowerheadroom',1,'upperheadroom',1,'headroomunit','bit','keepdatatype',1,'checkmin',0,'checkmax',0,'castoutput',0,'show',0),'gain',struct('variable','','description','','name','$S_$B_gain','width',1,'address','','max',NaN,'min',NaN,'class','default','type','CONTINUOUS','scaling','','lsb',1,'offset',0,'arb',0,'freeze',1,'unit','','keepdatatype',1,'value','1','scalar',0,'tolerance',1),'scalingvalid',0,'date',730486)  Gain=sqrt(3)/2  RndMeth=Zero
  Gain2 : Gain  Gain=0.5
  Gain3 : Gain  Tag=struct('comment',struct('text','','placement',1),'logdata',struct('maxnumvals',inf,'plotchannels',[],'loggingmode',3,'channels',1),'output',struct('variable','','description','','name','$S_$B','width',1,'address','','max',NaN,'min',NaN,'class','default','type','CONTINUOUS','scaling','','lsb',1,'offset',0,'arb',0,'freeze',1,'unit','','autoscalingmode',1,'lowerheadroom',1,'upperheadroom',1,'headroomunit','bit','keepdatatype',1,'checkmin',0,'checkmax',0,'castoutput',0,'show',0),'gain',struct('variable','','description','','name','$S_$B_gain','width',1,'address','','max',NaN,'min',NaN,'class','default','type','CONTINUOUS','scaling','','lsb',1,'offset',0,'arb',0,'freeze',1,'unit','','keepdatatype',1,'value','1','scalar',0,'tolerance',1),'scalingvalid',0,'date',730486)  Gain=1/2  RndMeth=Zero
  Gain4 : Gain  Gain=2/sqrt(3)
  MinMax1 : MinMax  SaturateOnIntegerOverflow=on  InputSameDT=on
  MinMax2 : MinMax  Function=max  SaturateOnIntegerOverflow=on  InputSameDT=on
  Mux4 : Mux  Inputs=3
  Sum2 : Sum  Inputs=--  RndMeth=Simplest
  Sum6 : Sum  Inputs=-+  RndMeth=Simplest
  V_phaA : Outport
  V_phaB : Outport  Port=2
  V_phaC : Outport  Port=3
  wires:
  Sum6/1 -> Sum2/2, Mux4/2
  Sum2/1 -> Mux4/3
  Gain1/1 -> Sum6/2
  Gain3/1 -> Sum6/1
  V_alpha/1 -> Gain3/1, Sum2/1, Mux4/1  "alpha"
  V_beta/1 -> Gain1/1  "beta"
  Add1/1 -> Gain4/1
  Add/1 -> Gain2/1
  Mux4/1 -> MinMax2/1, Add1/2, MinMax1/1
  MinMax1/1 -> Add/1
  MinMax2/1 -> Add/2
  Gain2/1 -> Add1/1
  Demux/1 -> V_phaA/1
  Demux/2 -> V_phaB/1
  Demux/3 -> V_phaC/1
  Gain4/1 -> Demux/1

== system BLDCmotorControl_FOC_R2017b/BLDC_controller/BLDC_controller/F03_Field_Oriented_Control/Inv_Park_Transform ==
  note: Inverse Park Transform:
      | V_alpha = V_d*cos(angle) - V_q*sin(angle)
      | V_beta = V_d*sin(angle) + V_q*cos(angle)
  V_q : Inport
  V_d : Inport  Port=2
  r_sin : Inport  Port=3
  r_cos : Inport  Port=4
  Divide{1..4} (4 alike) : Product  Inputs=**  OutDataTypeStr=Inherit: Inherit via back propagation  RndMeth=Simplest
  Sum1 : Sum  RndMeth=Simplest
  Sum6 : Sum  Inputs=+-  RndMeth=Simplest
  V_alpha : Outport
  V_beta : Outport  Port=2
  wires:
  r_sin/1 -> [r_sin]
  V_d/1 -> [V_d]
  V_q/1 -> [V_q]
  r_cos/1 -> [r_cos]
  [r_cos] -> Divide4/2
  [r_sin] -> Divide1/2
  [V_d] -> Divide4/1
  [r_cos] -> Divide3/2
  Divide1/1 -> Sum6/2
  [V_q] -> Divide1/1
  [V_d] -> Divide2/1
  Divide2/1 -> Sum1/1
  Divide3/1 -> Sum1/2
  [V_q] -> Divide3/1
  Divide4/1 -> Sum6/1
  [r_sin] -> Divide2/2
  Sum1/1 -> V_beta/1
  Sum6/1 -> V_alpha/1

== system BLDCmotorControl_FOC_R2017b/BLDC_controller/BLDC_controller/F03_Field_Oriented_Control/Outliers_Removal ==
  i_qRaw : Inport
  i_dRaw : Inport  Port=2
  i_DCLink : Inport  Port=3
  DCLink_Current_Available : Subsystem
  DCLink_Current_Not_Available : Subsystem
  If1 : If  IfExpression=u1 ~= 0
  Merge : Merge
  Merge1 : Merge
  b_DCLinkCurrAvail : Constant  Value=b_DCLinkCurrAvail  OutDataTypeStr=boolean
  i_q : Outport
  i_d : Outport  Port=2
  wires:
  [i_d] -> i_d/1
  [i_q] -> i_q/1
  i_qRaw/1 -> [i_qRaw]
  i_dRaw/1 -> [i_dRaw]
  [i_qRaw] -> DCLink_Current_Not_Available/1(i_qRaw)
  [i_dRaw] -> DCLink_Current_Not_Available/2(i_dRaw)
  If1/1 -> DCLink_Current_Available/Action
  i_DCLink/1 -> [i_DCLink]
  [i_dRaw] -> DCLink_Current_Available/2(i_dRaw)
  [i_qRaw] -> DCLink_Current_Available/1(i_qRaw)
  [i_DCLink] -> DCLink_Current_Available/3(i_DCLink)
  b_DCLinkCurrAvail/1 -> If1/1
  DCLink_Current_Not_Available/1(i_qNoDCLink) -> [i_qNoDCLink]
  DCLink_Current_Not_Available/2(i_dNoDCLink) -> [i_dNoDCLink]
  DCLink_Current_Available/1(i_qDCLink) -> [i_qDCLink]
  DCLink_Current_Available/2(i_dDCLink) -> [i_dDCLink]
  Merge1/1 -> [i_d]
  If1/2 -> DCLink_Current_Not_Available/Action
  [i_qNoDCLink] -> Merge/2
  [i_qDCLink] -> Merge/1
  [i_dDCLink] -> Merge1/1
  [i_dNoDCLink] -> Merge1/2
  Merge/1 -> [i_q]

== system BLDCmotorControl_FOC_R2017b/BLDC_controller/BLDC_controller/F03_Field_Oriented_Control/Park_Transform ==
  note: Park Transform:
      | i_q = -i_alpha*sin(angle) + i_beta*cos(angle)
      | i_d = i_alpha*cos(angle) + i_beta*sin(angle)
  i_apha : Inport
  i_beta : Inport  Port=2
  r_sin : Inport  Port=3
  r_cos : Inport  Port=4
  Divide{1..4} (4 alike) : Product  Inputs=**  OutDataTypeStr=Inherit: Inherit via back propagation  RndMeth=Simplest
  Sum1 : Sum  RndMeth=Simplest
  Sum6 : Sum  Inputs=-+  RndMeth=Simplest
  i_qRaw : Outport
  i_dRaw : Outport  Port=2
  wires:
  r_sin/1 -> [r_sin]
  i_beta/1 -> [i_beta]
  i_apha/1 -> [i_apha]
  r_cos/1 -> [r_cos]
  [r_sin] -> Divide4/2
  [i_apha] -> Divide4/1
  Divide4/1 -> Sum6/1
  Divide1/1 -> Sum6/2
  [i_beta] -> Divide1/1
  [r_cos] -> Divide1/2
  Sum6/1 -> i_qRaw/1
  Divide2/1 -> Sum1/1
  [i_apha] -> Divide2/1
  [r_cos] -> Divide2/2
  Divide3/1 -> Sum1/2
  [i_beta] -> Divide3/1
  [r_sin] -> Divide3/2
  Sum1/1 -> i_dRaw/1

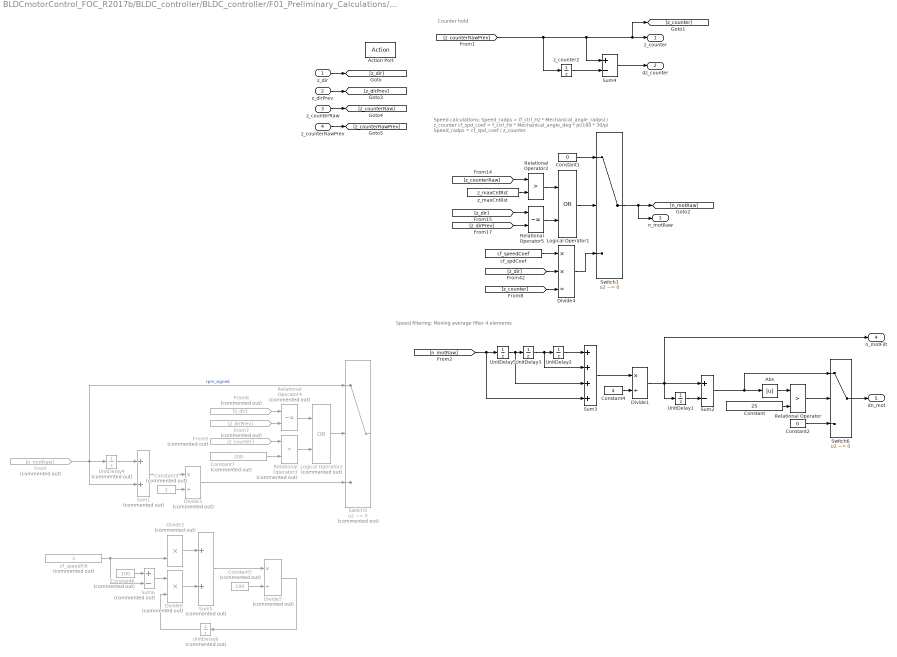
== system BLDCmotorControl_FOC_R2017b/BLDC_controller/BLDC_controller/F01_Preliminary_Calculations/F01_04_Speed_Calculation/Motor_Speed_Calculation ==
  note: Speed calculations:
      | Speed_radps = (f_ctrl_Hz * Mechanical_angle_radps) / z_counter
      | cf_spd_coef = f_ctrl_Hz * Mechanical_angle_deg * pi/180 * 30/pi
      | Speed_radps = cf_spd_coef / z_counter
  note: Speed filtering: Moving average filter 4 elements
  note: Counter hold
  z_dir : Inport
  z_dirPrev : Inport  Port=2
  z_counterRaw : Inport  Port=3
  z_counterRawPrev : Inport  Port=4
  Action Port : ActionPort  ActionType=then
  Abs : Abs
  Constant : Constant  Value=25  OutDataTypeStr=Inherit: Inherit via back propagation
  Constant1 : Constant  Value=0  OutDataTypeStr=Inherit: Inherit via back propagation
  Constant2 : Constant  Value=0  OutDataTypeStr=Inherit: Inherit via back propagation
  Constant3 : Constant  Commented=on  Value=2  OutDataTypeStr=Inherit: Inherit via back propagation
  Constant4 : Constant  Value=4  OutDataTypeStr=Inherit: Inherit via back propagation
  Constant5 : Constant  Commented=on  Value=100  OutDataTypeStr=Inherit: Inherit via back propagation
  Constant6 : Constant  Commented=on  Value=100  OutDataTypeStr=Inherit: Inherit via back propagation
  Constant7 : Constant  Commented=on  Value=200  OutDataTypeStr=Inherit: Inherit via back propagation
  Divide1 : Product  Inputs=*/  RndMeth=Simplest
  Divide2 : Product  Commented=on  Inputs=**  RndMeth=Simplest  OutDataTypeStr=Inherit: Same as first input
  Divide3 : Product  Commented=on  Inputs=*/  RndMeth=Simplest
  Divide4 : Product  Inputs=**/  RndMeth=Simplest  OutDataTypeStr=Inherit: Same as first input
  Divide5 : Product  Commented=on  Inputs=*/  RndMeth=Simplest  OutDataTypeStr=Inherit: Same as first input
  Divide6 : Product  Commented=on  Inputs=**  RndMeth=Simplest  OutDataTypeStr=Inherit: Same as first input
  From : From  Commented=on  GotoTag=n_motRaw
  From5 : From  Commented=on  GotoTag=z_counter
  From6 : From  Commented=on  GotoTag=z_dir
  From7 : From  Commented=on  GotoTag=z_dirPrev
  Logical Operator1 : Logic  Operator=OR  AllPortsSameDT=off  OutDataTypeStr=boolean
  Logical Operator2 : Logic  Commented=on  Operator=OR  AllPortsSameDT=off  OutDataTypeStr=boolean
  Relational Operator : RelationalOperator  Operator=>  OutDataTypeStr=boolean  RndMeth=Nearest
  Relational Operator2 : RelationalOperator  Operator=>  OutDataTypeStr=boolean  RndMeth=Simplest
  Relational Operator3 : RelationalOperator  Commented=on  Operator=>  OutDataTypeStr=boolean  RndMeth=Nearest
  Relational Operator4 : RelationalOperator  Commented=on  Operator=~=  OutDataTypeStr=boolean  RndMeth=Simplest
  Relational Operator5 : RelationalOperator  Operator=~=  OutDataTypeStr=boolean  RndMeth=Simplest
  Sum1 : Sum  Commented=on  RndMeth=Simplest  InputSameDT=on
  Sum2 : Sum  Inputs=+-  RndMeth=Simplest  InputSameDT=on  OutDataTypeStr=Inherit: Same as first input
  Sum3 : Sum  Inputs=++++  RndMeth=Simplest  InputSameDT=on
  Sum4 : Sum  Inputs=+-  RndMeth=Simplest  InputSameDT=on  OutDataTypeStr=Inherit: Same as first input
  Sum5 : Sum  Commented=on  RndMeth=Simplest  InputSameDT=on  OutDataTypeStr=Inherit: Same as first input
  Sum6 : Sum  Commented=on  Inputs=+-  RndMeth=Simplest  InputSameDT=on  OutDataTypeStr=Inherit: Same as first input
  Switch1 : Switch  Criteria=u2 ~= 0  OutDataTypeStr=Inherit: Inherit via back propagation  RndMeth=Zero
  Switch3 : Switch  Commented=on  Criteria=u2 ~= 0  OutDataTypeStr=Inherit: Inherit via back propagation  RndMeth=Zero
  Switch6 : Switch  Tag=struct('comment',struct('text','','placement',1),'logdata',struct('maxnumvals',inf,'plotchannels',[],'loggingmode',3,'channels',1),'output',struct('variable','','description','','name','$S_$B','width',1,'address','','max',NaN,'min',NaN,'class','default','type','CONTINUOUS','scaling','','lsb',1,'offset',0,'arb',0,'freeze',1,'unit','','autoscalingmode',1,'lowerheadroom',1,'upperheadroom',1,'headroomunit','bit','keepdatatype',1,'checkmin',0,'checkmax',0,'castoutput',0,'show',0),'threshold',struct('variable','','description','','name','$S_$B_threshold','width',1,'address','','max',NaN,'min',NaN,'class','default','type','CONTINUOUS','scaling','','lsb',1,'offset',0,'arb',0,'freeze',1,'unit','','keepdatatype',1,'value','0','scalar',0,'criteria',3),'scalingvalid',0,'date',733087.49614628474,'inheritscaling',0)  Criteria=u2 ~= 0  SaturateOnIntegerOverflow=on  InputSameDT=on
      settings: AttributesFormatString=threshold=%<threshold>\nCriteria : %<Criteria>
  UnitDelay{1..3,5} (4 alike) : UnitDelay  SampleTime=-1
  UnitDelay4 : UnitDelay  Commented=on  SampleTime=-1
  UnitDelay6 : UnitDelay  Commented=on  SampleTime=-1
  cf_spdCoef : Constant  Value=cf_speedCoef  OutDataTypeStr=int32
  cf_speedFilt : Constant  Commented=on  Value=3  OutDataTypeStr=int32
  z_counter2 : UnitDelay  InitialCondition=z_maxCntRst  SampleTime=-1
  z_maxCntRst : Constant  Value=z_maxCntRst  OutDataTypeStr=Inherit: Inherit via back propagation
  z_counter : Outport  InitialOutput=z_maxCntRst
  dz_counter : Outport  Port=2
  n_motRaw : Outport  Port=3
  n_motFilt : Outport  Port=4
  dn_mot : Outport  Port=5
  wires:
  [z_counterRawPrev] -> z_counter2/1, [z_counter], z_counter/1, Sum4/1
  z_counter2/1 -> Sum4/2
  [z_counter] -> Divide4/3
  [z_dir] -> Divide4/2
  cf_spdCoef/1 -> Divide4/1
  z_dir/1 -> [z_dir]
  From/1 -> Switch3/1, Sum1/2, UnitDelay4/1  "rpm_signed"
  UnitDelay4/1 -> Sum1/1
  Sum1/1 -> Divide3/1
  Constant3/1 -> Divide3/2
  [z_dirPrev] -> Relational Operator5/2
  Relational Operator2/1 -> Logical Operator1/1
  Logical Operator1/1 -> Switch1/2
  Relational Operator5/1 -> Logical Operator1/2
  Constant1/1 -> Switch1/1
  z_maxCntRst/1 -> Relational Operator2/2
  [z_counterRaw] -> Relational Operator2/1
  [z_dir] -> Relational Operator5/1
  z_counterRaw/1 -> [z_counterRaw]
  z_dirPrev/1 -> [z_dirPrev]
  z_counterRawPrev/1 -> [z_counterRawPrev]
  UnitDelay1/1 -> Sum2/2
  Relational Operator/1 -> Switch6/2
  Constant2/1 -> Switch6/3
  Abs/1 -> Relational Operator/1
  Constant/1 -> Relational Operator/2
  Switch1/1 -> n_motRaw/1, [n_motRaw]
  Divide4/1 -> Switch1/3
  Sum4/1 -> dz_counter/1
  From5/1 -> Relational Operator3/1
  Constant7/1 -> Relational Operator3/2
  Logical Operator2/1 -> Switch3/2
  Relational Operator3/1 -> Logical Operator2/2
  From6/1 -> Relational Operator4/1
  From7/1 -> Relational Operator4/2
  Relational Operator4/1 -> Logical Operator2/1
  Divide3/1 -> Switch3/3
  Divide1/1 -> n_motFilt/1, Sum2/1, UnitDelay1/1
  Constant4/1 -> Divide1/2
  Sum3/1 -> Divide1/1
  UnitDelay2/1 -> Sum3/1
  UnitDelay3/1 -> Sum3/2, UnitDelay2/1
  UnitDelay5/1 -> Sum3/3, UnitDelay3/1
  [n_motRaw] -> Sum3/4, UnitDelay5/1
  UnitDelay6/1 -> Divide6/2
  Sum5/1 -> Divide5/1
  Constant6/1 -> Sum6/1
  Divide6/1 -> Sum5/2
  Sum6/1 -> Divide6/1
  cf_speedFilt/1 -> Divide2/2, Sum6/2
  Constant5/1 -> Divide5/2
  Divide5/1 -> UnitDelay6/1
  Divide2/1 -> Sum5/1
  Switch6/1 -> dn_mot/1
  Sum2/1 -> Switch6/1, Abs/1
